simulink library "VCTlbx"  (R2018b)
settings: Solver=VariableStepAuto  StartTime=0.0  StopTime=10.0  RelTol=1e-3  EnableMultiTasking=on
undefined symbols (not defined in the file or in its folder): prefix, suffix
libraries: commrandsrc3 x3, powerlib_meascontrol x2, $bdroot x2, simulink x1
settings Model: Creator=Ulysses  LastModifiedBy=bernardu
settings DataIOCC: LimitDataPoints=on
settings OptimizationCC: LifeSpan=inf
settings DebuggingCC: AllowSymbolicDim=off  SFUnexpectedBacktrackingDiag=warning  SFNoUnconditionalDefaultTransitionDiag=warning
settings ModelReferenceCC: PropagateSignalLabelsOutOfModel=off
settings SFSimCC: SimUseLocalCustomCode=off
settings RTWCC: RTWUseLocalCustomCode=off
settings CodeAppCC: StateflowObjectComments=on
settings GRTTargetCC: TargetLangStandard=C89/C90 (ANSI)
settings ConfigComp: CovMetricSettings=dw  CovHtmlReporting=on  CovSaveCumulativeToWorkspaceVar=on  CovSaveSingleToWorkspaceVar=on  CovExternalEMLEnable=off

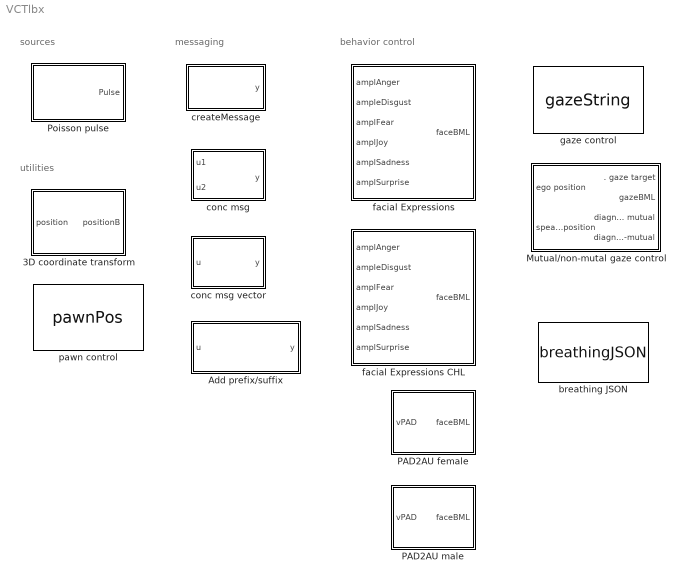
== system VCTlbx ==
  note: utilities
  note: sources
  note: behavior control
  note: messaging
  3D coordinate transform : Subsystem  mask(3D coordinate transform){zeroA=[], zeroB=[], minmaxXA=[], minmaxXB=[], minmaxYA=[], minmaxYB=[], minmaxZA=[], minmaxZB=[]}
      mask prompts: zeroA "center point input [3D]"; zeroB "center point output [3D]"; minmaxXA "min/max X input [2D]"; minmaxXB "min/max X output [2D]"; minmaxYA "min/max Y input [2D]"; minmaxYB "min/max Y output [2D]"; minmaxZA "min/max Z input [2D]"; minmaxZB "min/max Z output [2D]"
      mask help: Transform 3D coordinates from scale and center to another.
      mask TypeOptions zeroA: zeroA/zeroA
      mask TypeOptions zeroB: zeroB/zeroB
      mask TypeOptions minmaxXA: minmaxXA/minmaxXA
      mask TypeOptions minmaxXB: minmaxXB/minmaxXB
      mask TypeOptions minmaxYA: minmaxYA/minmaxYA
      mask TypeOptions minmaxYB: minmaxYB/minmaxYB
      mask TypeOptions minmaxZA: minmaxZA/minmaxZA
      mask TypeOptions minmaxZB: minmaxZB/minmaxZB
  Add prefix/suffix : MATLAB Function  TreatAsAtomicUnit=on  mask(Prefix/suffix message){paramPrefix=<?xml version="1.0" ?><act><bml>, paramSuffix=</bml></act>}
  Mutual/non-mutal gaze control : Subsystem  Description=|  mask(Mutual/non-mutal randomized gaze){PoissonParameterMutual=5, PoissonParameterNonMutual=5, paramVarianceVertical=pi/10, paramExtent=.3, paramVarianceHorizontal=pi/2}
      | this block implements an oscillation between two Poisson processes; one for mutual and 
      | one for non-mutual gaze
      mask prompts: PoissonParameterMutual "Poisson parameter (Lambda) for mutual gaze:"; PoissonParameterNonMutual "Poisson parameter (Lambda) for non-mutual gaze:"; paramVarianceVertical "Variance vertical"; paramExtent "Extent [0...1]"; paramVarianceHorizontal "Variance horizontal"
      mask help:
      | this block implements an oscillation between two Poisson processes; one for mutual and
      | one for non-mutual gaze
      mask TypeOptions PoissonParameterMutual: Poisson social Gaze/PoissonParameterMutual
      mask TypeOptions PoissonParameterNonMutual: Poisson social Gaze/PoissonParameterNonMutual
      mask TypeOptions paramVarianceVertical: randomGaze1/RN vert/Variance
      mask TypeOptions paramExtent: Extent/Value
      mask TypeOptions paramVarianceHorizontal: randomGaze1/RN horiz/Variance
  PAD2AU female : Subsystem  mask(PAD to face BML (female)){gainAU_1=[-0.086 -0.001 -0.062], gainAU_2=[0.015 +0.018 +0.104], gainAU_4=[-0.067 -0.017 +0.078], gainAU_5=[0.003 +0.120 -0.017], gainAU_6=[-0.009 -0.012 +0.036], gainAU_7=[0.004 -0.021 +0.040], gainAU_9=[-0.007 +0.001 +0.086], gainAU_10=[-0.089 -0.007 +0.028], gainAU_11=[0.000 -0.017 +0.028], gainAU_12=[0.114 -0.009 +0.013], gainAU_13=[0.063 -0.011 +0.033], gainAU_14=[0.049 -0.025 +0.054], gainAU_15=[-0.073 -0.008 +0.035], gainAU_16=[-0.048 +0.049 +0.006], gainAU_17=[-0.071 -0.005 +0.023], gainAU_18=[0.013 -0.033 +0.041], gainAU_20=[-0.009 -0.010 +0.029], gainAU_22=[0.057 +0.013 -0.002], gainAU_23=[0.009 -0.007 +0.050], gainAU_24=[-0.016 -0.042 +0.041], gainAU_25=[0.157 +0.100 +0.095], gainAU_26=[0.041 -0.022 +0.081], gainAU_27=[0.060 +0.079 +0.127], gainAD_28=[0.017 -0.031 +0.052], gainAD_29=[-0.001 -0.010 +0.051], gainAU_30=[-0.005 -0.003 -0.004], gainAU_31=[-0.016 +0.013 +0.052], gainAU_32=[-0.012 -0.044 +0.006], gainAU_33=[-0.017 -0.006 +0.032], gainAD_34=[0.009 -0.028 +0.035], gainAD_35=[0.000 -0.019 +0.044], gainAU_38=[-0.023 -0.018 +0.050], gainAU_39=[-0.004 -0.024 +0.034], gainAU_43=[-0.019 -0.131 +0.076]}
      mask prompts: gainAU_1 "gain for AU_1"; gainAU_2 "gain for AU_2"; gainAU_4 "gain for AU_4"; gainAU_5 "gain for AU_5"; gainAU_6 "gain for AU_6"; gainAU_7 "gain for AU_7"; gainAU_9 "gain for AU_9"; gainAU_10 "gain for AU_10"; gainAU_11 "gain for AU_11"; gainAU_12 "gain for AU_12"; gainAU_13 "gain for AU_13"; gainAU_14 "gain for AU_14"; gainAU_15 "gain for AU_15"; gainAU_16 "gain for AU_16"; gainAU_17 "gain for AU_17"; gainAU_18 "gain for AU_18"; gainAU_20 "gain for AU_20"; gainAU_22 "gain for AU_22"; gainAU_23 "gain for AU_23"; gainAU_24 "gain for AU_24"; gainAU_25 "gain for AU_25"; gainAU_26 "gain for AU_26"; gainAU_27 "gain for AU_27"; gainAD_28 "gain for AD_28"; gainAD_29 "gain for AD_29"; gainAU_30 "gain for AU_30"; gainAU_31 "gain for AU_31"; gainAU_32 "gain for AU_32"; gainAU_33 "gain for AU_33"; gainAD_34 "gain for AD_34"; gainAD_35 "gain for AD_35"; gainAU_38 "gain for AU_38"; gainAU_39 "gain for AU_39"; gainAU_43 "gain for AU_43"
      mask help:
      | Creates a BML message from Pleasure Arousal Dominance input. Mappings are based on:
      | Hana Boukricha, Ipke Wachsmuth, Andrea Hofstatter, and Karl Grammer. 2009. Pleasure-arousal-dominance driven facial expression simulation. 2009 3rd International Conference on Affective Computing and Intelligent Interaction and Workshops, IEEE, 1–7. http://doi.org/10.1109/ACII.2009.5349579
      mask TypeOptions gainAU_1: gainAU_1/Gain
      mask TypeOptions gainAU_2: gainAU_2/Gain
      mask TypeOptions gainAU_4: gainAU_4/Gain
      mask TypeOptions gainAU_5: gainAU_5/Gain
      mask TypeOptions gainAU_6: gainAU_6/Gain
      mask TypeOptions gainAU_7: gainAU_7/Gain
      mask TypeOptions gainAU_9: gainAU_9/Gain
      mask TypeOptions gainAU_10: gainAU_10/Gain
      mask TypeOptions gainAU_11: gainAU_11/Gain
      mask TypeOptions gainAU_12: gainAU_12/Gain
      mask TypeOptions gainAU_13: gainAU_13/Gain
      mask TypeOptions gainAU_14: gainAU_14/Gain
      mask TypeOptions gainAU_15: gainAU_15/Gain
      mask TypeOptions gainAU_16: gainAU_16/Gain
      mask TypeOptions gainAU_17: gainAU_17/Gain
      mask TypeOptions gainAU_18: gainAU_18/Gain
      mask TypeOptions gainAU_20: gainAU_20/Gain
      mask TypeOptions gainAU_22: gainAU_22/Gain
      mask TypeOptions gainAU_23: gainAU_23/Gain
      mask TypeOptions gainAU_24: gainAU_24/Gain
      mask TypeOptions gainAU_25: gainAU_25/Gain
      mask TypeOptions gainAU_26: gainAU_26/Gain
      mask TypeOptions gainAU_27: gainAU_27/Gain
      mask TypeOptions gainAD_28: gainAD_28/Gain
      mask TypeOptions gainAD_29: gainAD_29/Gain
      mask TypeOptions gainAU_30: gainAU_30/Gain
      mask TypeOptions gainAU_31: gainAU_31/Gain
      mask TypeOptions gainAU_32: gainAU_32/Gain
      mask TypeOptions gainAU_33: gainAU_33/Gain
      mask TypeOptions gainAD_34: gainAD_34/Gain
      mask TypeOptions gainAD_35: gainAD_35/Gain
      mask TypeOptions gainAU_38: gainAU_38/Gain
      mask TypeOptions gainAU_39: gainAU_39/Gain
      mask TypeOptions gainAU_43: gainAU_43/Gain
  PAD2AU male : Subsystem  mask(PAD to face BML (male)){gainAU_1=[0.003 -0.002 -0.016 ], gainAU_2=[-0.002 +0.010 -0.030], gainAU_27=[-0.016 +0.034 +0.019], gainAU_26=[-0.002 +0.049 -0.006], gainAU_6=[-0.008 +0.009 +0.004], gainAU_18=[0.002 +0.004 +0.014 ], gainAU_22=[0.007 +0.025 +0.006 ], gainAU_14=[0.003 +0.009 -0.002 ], gainAU_17=[-0.010 +0.017 +0.000], gainAU_10=[-0.053 +0.026 +0.014], gainAU_5=[-0.003 +0.032 -0.000], gainAU_43=[-0.021 -0.037 -0.011], gainAU_4=[-0.036 +0.022 +0.019], gainAU_9=[-0.008 +0.006 +0.005], gainAU_39=[-0.004 +0.004 -0.008], gainAU_38=[-0.010 +0.008 +0.005], gainAU_25=[-0.023 +0.058 +0.008], gainAU_24=[-0.004 -0.003 -0.007], gainAU_23=[-0.011 +0.009 -0.007], gainAU_19=[-0.004 +0.003 +0.001], gainAU_13=[0.039 +0.015 -0.004 ], gainAU_7=[-0.005 -0.001 +0.009], gainAU_12=[0.057 +0.009 -0.019 ], gainAU_11=[-0.008 +0.009 +0.001], gainAU_15=[-0.046 -0.002 -0.003], gainAU_16=[-0.014 +0.016 -0.002], gainAU_20=[-0.026 +0.010 -0.002]}
      mask prompts: gainAU_1 "gain for AU_1"; gainAU_2 "gain for AU_2"; gainAU_27 "gain for AU_27"; gainAU_26 "gain for AU_26"; gainAU_6 "gain for AU_6"; gainAU_18 "gain for AU_18"; gainAU_22 "gain for AU_22"; gainAU_14 "gain for AU_14"; gainAU_17 "gain for AU_17"; gainAU_10 "gain for AU_10"; gainAU_5 "gain for AU_5"; gainAU_43 "gain for AU_43"; gainAU_4 "gain for AU_4"; gainAU_9 "gain for AU_9"; gainAU_39 "gain for AU_39"; gainAU_38 "gain for AU_38"; gainAU_25 "gain for AU_25"; gainAU_24 "gain for AU_24"; gainAU_23 "gain for AU_23"; gainAU_19 "gain for AU_19"; gainAU_13 "gain for AU_13"; gainAU_7 "gain for AU_7"; gainAU_12 "gain for AU_12"; gainAU_11 "gain for AU_11"; gainAU_15 "gain for AU_15"; gainAU_16 "gain for AU_16"; gainAU_20 "gain for AU_20"
      mask help:
      | Creates a BML message from Pleasure Arousal Dominance input. Mappings are based on:
      | Hana Boukricha, Ipke Wachsmuth, Andrea Hofstatter, and Karl Grammer. 2009. Pleasure-arousal-dominance driven facial expression simulation. 2009 3rd International Conference on Affective Computing and Intelligent Interaction and Workshops, IEEE, 1–7. http://doi.org/10.1109/ACII.2009.5349579
      mask TypeOptions gainAU_1: gainAU_1/Gain
      mask TypeOptions gainAU_2: gainAU_2/Gain
      mask TypeOptions gainAU_27: gainAU_27/Gain
      mask TypeOptions gainAU_26: gainAU_26/Gain
      mask TypeOptions gainAU_6: gainAU_6/Gain
      mask TypeOptions gainAU_18: gainAU_18/Gain
      mask TypeOptions gainAU_22: gainAU_22/Gain
      mask TypeOptions gainAU_14: gainAU_14/Gain
      mask TypeOptions gainAU_17: gainAU_17/Gain
      mask TypeOptions gainAU_10: gainAU_10/Gain
      mask TypeOptions gainAU_5: gainAU_5/Gain
      mask TypeOptions gainAU_43: gainAU_43/Gain
      mask TypeOptions gainAU_4: gainAU_4/Gain
      mask TypeOptions gainAU_9: gainAU_9/Gain
      mask TypeOptions gainAU_39: gainAU_39/Gain
      mask TypeOptions gainAU_38: gainAU_38/Gain
      mask TypeOptions gainAU_25: gainAU_25/Gain
      mask TypeOptions gainAU_24: gainAU_24/Gain
      mask TypeOptions gainAU_23: gainAU_23/Gain
      mask TypeOptions gainAU_19: gainAU_19/Gain
      mask TypeOptions gainAU_13: gainAU_13/Gain
      mask TypeOptions gainAU_7: gainAU_7/Gain
      mask TypeOptions gainAU_12: gainAU_12/Gain
      mask TypeOptions gainAU_11: gainAU_11/Gain
      mask TypeOptions gainAU_15: gainAU_15/Gain
      mask TypeOptions gainAU_16: gainAU_16/Gain
      mask TypeOptions gainAU_20: gainAU_20/Gain
  Poisson pulse : Subsystem  mask(Poisson pulse){PoissonParameter=3}
      mask prompts: PoissonParameter "Poisson parameter (Lambda):"
      mask help: Generates a pulse train with Poisson distributed delays.
      mask TypeOptions PoissonParameter: triggered Poisson/Poisson numbers/PoissonParameter
  breathing JSON : S-Function  FunctionName=breathingJSON  Parameters=double(charname)  SFunctionDeploymentMode=off  EnableBusSupport=off  mask(Send JSON formatted breathing blendshape control){charname='FuseCharacter'}
      mask prompts: charname "Character Name"
      mask help:
      | Send JSON with the following format:
      | {
      |    "blendshape_ctrl":{
      |       "blendshapes_names":[
      |          "Tops_BreatheChest",
      |          "Tops_BreatheStomach"
      |       ],
      |       "blendshapes_weights":[
      |          <thx>,
      |          <abd>
      |       ],
      |       "mesh":"Tops"
      |    },
      |    "character":"FuseCharacter",
      |    "joint_rotation":{
      |       "name":"Hips/Spine/Spine1/Spine2/Neck/Head",
      |       "quaternion":[
      |          <x>,
      |          <y>,
      |          <z>,
      |          <w>
      |       ]
      |    }
      | }
      mask Display:
      | port_label('input', 1, 'thx')
      | port_label('input', 2, 'abd')
      | port_label('input', 3, 'neck')
      | port_label('output', 1, 'JSON')
      | disp('{}')
  conc msg : MATLAB Function  TreatAsAtomicUnit=on  mask(Concatenate messages){}
      mask help: Concatenates all messages (represented as double arrays) into a single one. Max length of concatenated message is 2048.
  conc msg vector : MATLAB Function  TreatAsAtomicUnit=on  mask(Concatenate messages){}
      mask help: Concatenates all messages (represented as double arrays) into a single one. Max length of concatenated message is 2048.
  createMessage : MATLAB Function  TreatAsAtomicUnit=on  mask(createMessage){paramMessage=message}
      mask prompts: paramMessage "Message"
      mask help: Create double array message from input string. Max length = 2048. DO NOT USE QUOTES
  facial Expressions : Subsystem  mask(Categorical facial experssions){}
      mask help: Block to generate categorical facial expressions. Input is amplitude [0...1].
      mask Display:
      | port_label('input', 1, 'ampl. Anger');
      | port_label('input', 2, 'ampl. Disgust');
      | port_label('input', 3, 'ampl. Fear');
      | port_label('input', 4, 'ampl. Joy');
      | port_label('input', 5, 'ampl. Sadness');
      | port_label('input', 6, 'ampl. Surprise');
      | port_label('output', 1, 'faceBML');
  facial Expressions CHL : Subsystem  AncestorBlock=VCTlbx/facial Expressions  mask(Categorical facial experssions){}
      mask help: Block to generate categorical facial expressions. Input is amplitude [0...1].
      mask Display:
      | port_label('input', 1, 'ampl. Anger');
      | port_label('input', 2, 'ampl. Disgust');
      | port_label('input', 3, 'ampl. Fear');
      | port_label('input', 4, 'ampl. Joy');
      | port_label('input', 5, 'ampl. Sadness');
      | port_label('input', 6, 'ampl. Surprise');
      | port_label('output', 1, 'faceBML');
  gaze control : S-Function  FunctionName=gazeString  SFunctionDeploymentMode=off  EnableBusSupport=off  mask(gaze BML){}
      mask Display:
      | port_label('input', 1, 'xpos')
      | port_label('input', 2, 'ypos')
      | port_label('input', 3, 'zpos')
      | port_label('input', 4, 'extent')
      | port_label('output', 1, 'gaze BML')
  pawn control : S-Function  FunctionName=pawnPos  SFunctionDeploymentMode=off  EnableBusSupport=off
      mask Display:
      | port_label('input', 1, 'xpos')
      | port_label('input', 2, 'ypos')
      | port_label('input', 3, 'zpos')
      | port_label('output', 1, 'pawn SBM')

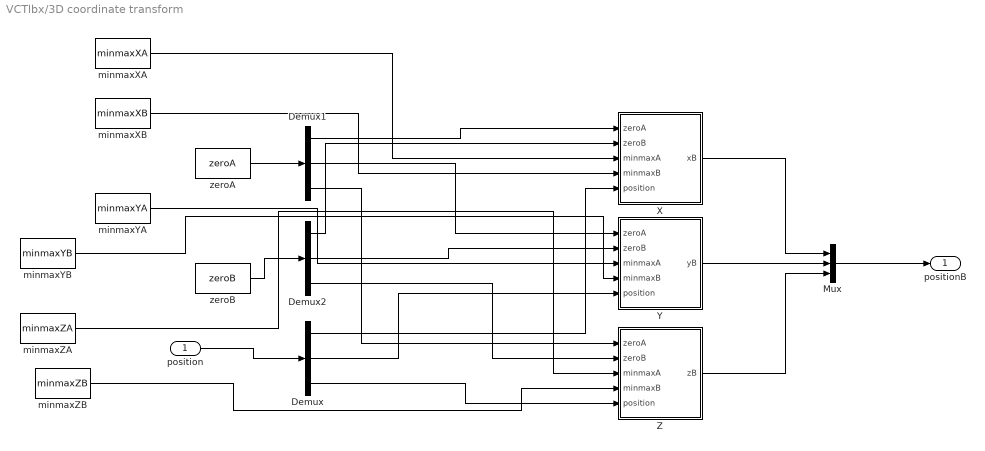
== system VCTlbx/3D coordinate transform ==
  position : Inport  PortDimensions=3
  Demux : Demux  Outputs=3
  Demux1 : Demux  Outputs=3
  Demux2 : Demux  Outputs=3
  Mux : Mux  Inputs=3
  X : Subsystem
  Y : Subsystem
  Z : Subsystem
  minmaxXA : Constant  Value=minmaxXA  VectorParams1D=off  mask{minmaxXA=minmaxXA}
      mask prompts: minmaxXA "min/max X input [2D]"
  minmaxXB : Constant  Value=minmaxXB  VectorParams1D=off  mask{minmaxXB=minmaxXB}
      mask prompts: minmaxXB "min/max X output [2D]"
  minmaxYA : Constant  Value=minmaxYA  VectorParams1D=off  mask{minmaxYA=minmaxYA}
      mask prompts: minmaxYA "min/max Y input [2D]"
  minmaxYB : Constant  Value=minmaxYB  VectorParams1D=off  mask{minmaxYB=minmaxYB}
      mask prompts: minmaxYB "min/max Y output [2D]"
  minmaxZA : Constant  Value=minmaxZA  VectorParams1D=off  mask{minmaxZA=minmaxZA}
      mask prompts: minmaxZA "min/max Z input [2D]"
  minmaxZB : Constant  Value=minmaxZB  VectorParams1D=off  mask{minmaxZB=minmaxZB}
      mask prompts: minmaxZB "min/max Z output [2D]"
  zeroA : Constant  Value=zeroA  VectorParams1D=off  mask{zeroA=zeroA}
      mask prompts: zeroA "center point input [3D]"
  zeroB : Constant  Value=zeroB  VectorParams1D=off  mask{zeroB=zeroB}
      mask prompts: zeroB "center point output [3D]"
  positionB : Outport
  wires:
  Demux/1 -> X/5(position)
  Demux1/3 -> Z/1(zeroA)
  Demux1/2 -> Y/1(zeroA)
  Demux2/1 -> X/2(zeroB)
  X/1(xB) -> Mux/1
  Demux/3 -> Z/5(position)
  Demux1/1 -> X/1(zeroA)
  position/1 -> Demux/1
  Demux/2 -> Y/5(position)
  Y/1(yB) -> Mux/2
  minmaxXA/1 -> X/3(minmaxA)
  Z/1(zB) -> Mux/3
  minmaxYB/1 -> Y/4(minmaxB)
  minmaxXB/1 -> X/4(minmaxB)
  Mux/1 -> positionB/1
  Demux2/3 -> Z/2(zeroB)
  zeroA/1 -> Demux1/1
  zeroB/1 -> Demux2/1
  minmaxZB/1 -> Z/4(minmaxB)
  Demux2/2 -> Y/2(zeroB)
  minmaxYA/1 -> Y/3(minmaxA)
  minmaxZA/1 -> Z/3(minmaxA)

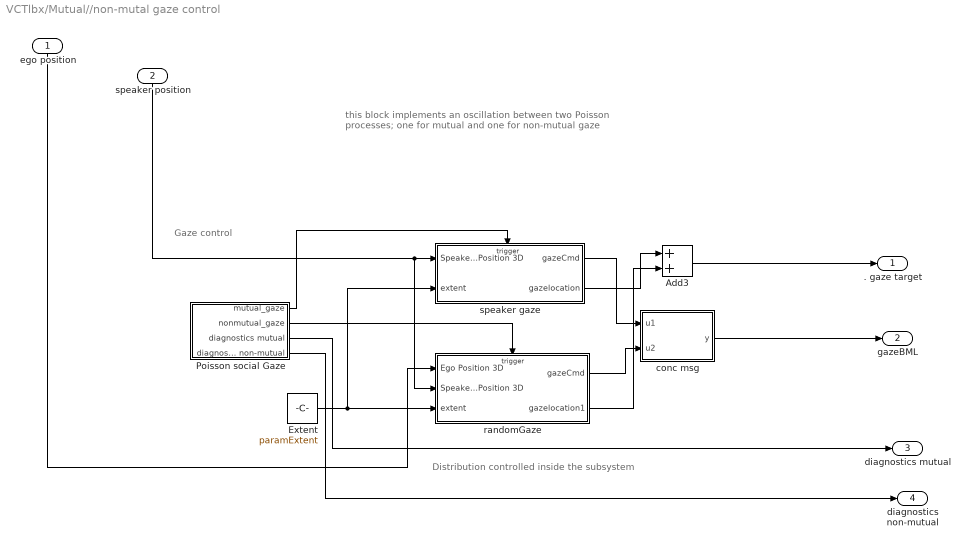
== system VCTlbx/Mutual//non-mutal gaze control ==
  note: Gaze control
  note: Distribution controlled inside the subsystem
  note: this block implements an oscillation
      | between two Poisson processes; one for mutual and
      | one for non-mutual gaze
  ego position : Inport
  speaker position : Inport  Port=2
  Add3 : Sum
  Extent : Constant  Value=paramExtent
  Poisson social Gaze : Subsystem  mask(Poisson pulse){PoissonParameterMutual=PoissonParameterMutual, PoissonParameterNonMutual=PoissonParameterNonMutual}
      mask prompts: PoissonParameterMutual "Poisson parameter (Lambda) for mutual gaze:"; PoissonParameterNonMutual "Poisson parameter (Lambda) for non-mutual gaze:"
      mask help: Generates a pulse train with Poisson distributed delays.
      mask TypeOptions PoissonParameterMutual: p mutual/Poisson numbers mutual/PoissonParameter
      mask TypeOptions PoissonParameterNonMutual: p nonmutual/Poisson numbers nonmutual/PoissonParameter
  conc msg : MATLAB Function  TreatAsAtomicUnit=on  mask(Concatenate messages){}
      mask help: Concatenates all messages (represented as double arrays) into a single one. Max length of concatenated message is 2048.
  randomGaze : Subsystem  TreatAsAtomicUnit=on
  speaker gaze : Subsystem  TreatAsAtomicUnit=on
  . gaze target : Outport
  gazeBML : Outport  Port=2
  diagnostics mutual : Outport  Port=3
  diagnostics non-mutual : Outport  Port=4
  wires:
  Poisson social Gaze/4(diagnostics non-mutual) -> diagnostics non-mutual/1
  Poisson social Gaze/3(diagnostics mutual) -> diagnostics mutual/1
  Add3/1 -> . gaze target/1
  Extent/1 -> randomGaze/3(extent), speaker gaze/2(extent)
  speaker gaze/2(gazelocation) -> Add3/1
  Poisson social Gaze/2(nonmutual_gaze) -> randomGaze/Trigger
  ego position/1 -> randomGaze/1(Ego Position 3D)
  randomGaze/1(gazeCmd) -> conc msg/2(u2)
  randomGaze/2(gazelocation1) -> Add3/2
  speaker position/1 -> speaker gaze/1("Speaker Position 3D "), randomGaze/2("Speaker Position 3D ")
  speaker gaze/1(gazeCmd) -> conc msg/1(u1)
  Poisson social Gaze/1(mutual_gaze) -> speaker gaze/Trigger
  conc msg/1(y) -> gazeBML/1

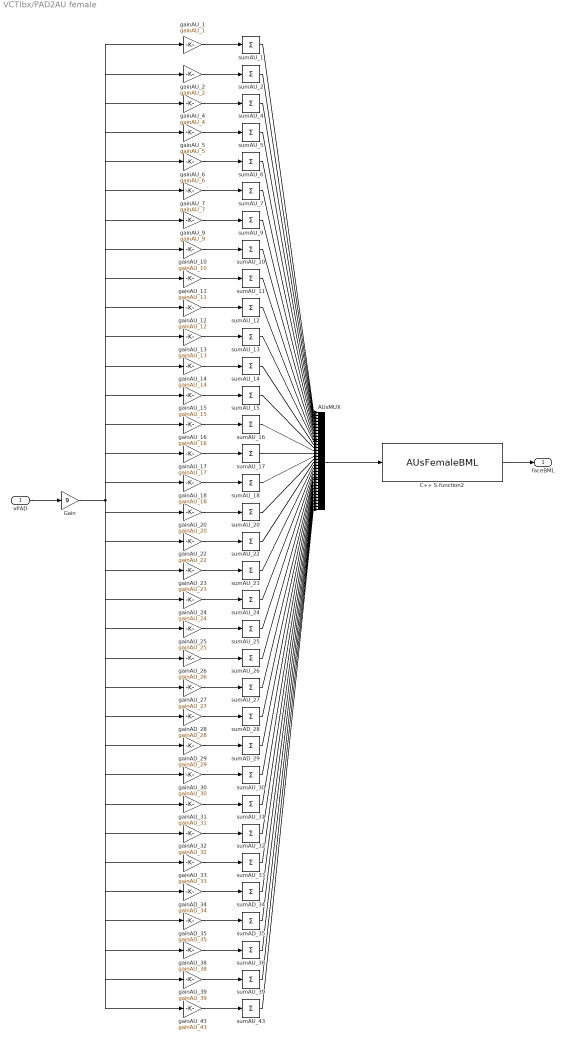
== system VCTlbx/PAD2AU female ==
  vPAD : Inport
  AUsMUX : Mux  Inputs=34
  C++ S-function2 : S-Function  FunctionName=AUsFemaleBML  SFunctionDeploymentMode=off  EnableBusSupport=off
  Gain : Gain  Gain=9
  gainAD_28 : Gain  Gain=gainAD_28
  gainAD_29 : Gain  Gain=gainAD_29
  gainAD_34 : Gain  Gain=gainAD_34
  gainAD_35 : Gain  Gain=gainAD_35
  gainAU_1 : Gain  Gain=gainAU_1
  gainAU_10 : Gain  Gain=gainAU_10
  gainAU_11 : Gain  Gain=gainAU_11
  gainAU_12 : Gain  Gain=gainAU_12
  gainAU_13 : Gain  Gain=gainAU_13
  gainAU_14 : Gain  Gain=gainAU_14
  gainAU_15 : Gain  Gain=gainAU_15
  gainAU_16 : Gain  Gain=gainAU_16
  gainAU_17 : Gain  Gain=gainAU_17
  gainAU_18 : Gain  Gain=gainAU_18
  gainAU_2 : Gain  Gain=gainAU_2
  gainAU_20 : Gain  Gain=gainAU_20
  gainAU_22 : Gain  Gain=gainAU_22
  gainAU_23 : Gain  Gain=gainAU_23
  gainAU_24 : Gain  Gain=gainAU_24
  gainAU_25 : Gain  Gain=gainAU_25
  gainAU_26 : Gain  Gain=gainAU_26
  gainAU_27 : Gain  Gain=gainAU_27
  gainAU_30 : Gain  Gain=gainAU_30
  gainAU_31 : Gain  Gain=gainAU_31
  gainAU_32 : Gain  Gain=gainAU_32
  gainAU_33 : Gain  Gain=gainAU_33
  gainAU_38 : Gain  Gain=gainAU_38
  gainAU_39 : Gain  Gain=gainAU_39
  gainAU_4 : Gain  Gain=gainAU_4
  gainAU_43 : Gain  Gain=gainAU_43
  gainAU_5 : Gain  Gain=gainAU_5
  gainAU_6 : Gain  Gain=gainAU_6
  gainAU_7 : Gain  Gain=gainAU_7
  gainAU_9 : Gain  Gain=gainAU_9
  sumAD_{28..29,34..35} (4 alike) : Sum  Inputs=+
  sumAU_{1..2,4..7,9..18,20,22..27,30..33,38..39,43} (30 alike) : Sum  Inputs=+
  faceBML : Outport
  wires:
  AUsMUX/1 -> C++ S-function2/1
  sumAU_6/1 -> AUsMUX/5
  gainAU_6/1 -> sumAU_6/1
  gainAU_7/1 -> sumAU_7/1
  sumAU_9/1 -> AUsMUX/7
  gainAU_9/1 -> sumAU_9/1
  sumAU_7/1 -> AUsMUX/6
  gainAU_10/1 -> sumAU_10/1
  sumAU_10/1 -> AUsMUX/8
  sumAU_14/1 -> AUsMUX/12
  gainAU_15/1 -> sumAU_15/1
  sumAU_15/1 -> AUsMUX/13
  gainAU_14/1 -> sumAU_14/1
  sumAU_16/1 -> AUsMUX/14
  gainAU_17/1 -> sumAU_17/1
  gainAU_16/1 -> sumAU_16/1
  sumAU_4/1 -> AUsMUX/3
  sumAU_2/1 -> AUsMUX/2
  gainAU_2/1 -> sumAU_2/1
  gainAU_4/1 -> sumAU_4/1
  sumAU_5/1 -> AUsMUX/4
  gainAU_5/1 -> sumAU_5/1
  gainAU_11/1 -> sumAU_11/1
  sumAU_11/1 -> AUsMUX/9
  gainAU_13/1 -> sumAU_13/1
  gainAU_12/1 -> sumAU_12/1
  sumAU_12/1 -> AUsMUX/10
  sumAU_13/1 -> AUsMUX/11
  sumAU_18/1 -> AUsMUX/16
  sumAU_17/1 -> AUsMUX/15
  gainAU_18/1 -> sumAU_18/1
  gainAU_20/1 -> sumAU_20/1
  sumAU_22/1 -> AUsMUX/18
  sumAU_20/1 -> AUsMUX/17
  gainAU_22/1 -> sumAU_22/1
  gainAU_23/1 -> sumAU_23/1
  sumAU_23/1 -> AUsMUX/19
  gainAU_24/1 -> sumAU_24/1
  sumAU_25/1 -> AUsMUX/21
  gainAU_26/1 -> sumAU_26/1
  gainAU_25/1 -> sumAU_25/1
  sumAU_24/1 -> AUsMUX/20
  gainAD_28/1 -> sumAD_28/1
  sumAU_26/1 -> AUsMUX/22
  gainAU_27/1 -> sumAU_27/1
  sumAU_27/1 -> AUsMUX/23
  sumAD_29/1 -> AUsMUX/25
  sumAD_28/1 -> AUsMUX/24
  gainAD_29/1 -> sumAD_29/1
  sumAU_31/1 -> AUsMUX/27
  sumAU_30/1 -> AUsMUX/26
  gainAU_31/1 -> sumAU_31/1
  gainAU_30/1 -> sumAU_30/1
  sumAU_32/1 -> AUsMUX/28
  gainAU_32/1 -> sumAU_32/1
  gainAU_33/1 -> sumAU_33/1
  sumAU_33/1 -> AUsMUX/29
  gainAD_34/1 -> sumAD_34/1
  sumAD_35/1 -> AUsMUX/31
  gainAU_38/1 -> sumAU_38/1
  gainAD_35/1 -> sumAD_35/1
  sumAU_38/1 -> AUsMUX/32
  sumAD_34/1 -> AUsMUX/30
  gainAU_39/1 -> sumAU_39/1
  sumAU_39/1 -> AUsMUX/33
  gainAU_43/1 -> sumAU_43/1
  sumAU_43/1 -> AUsMUX/34
  sumAU_1/1 -> AUsMUX/1
  Gain/1 -> gainAU_1/1, gainAU_2/1, gainAU_4/1, gainAU_5/1, gainAU_6/1, gainAU_7/1, gainAU_9/1, gainAU_10/1, gainAU_11/1, gainAU_12/1, gainAU_13/1, gainAU_14/1, gainAU_15/1, gainAU_16/1, gainAU_17/1, gainAU_18/1, gainAU_20/1, gainAU_22/1, gainAU_23/1, gainAU_24/1, gainAU_25/1, gainAU_26/1, gainAU_27/1, gainAD_28/1, gainAD_29/1, gainAU_30/1, gainAU_31/1, gainAU_32/1, gainAU_33/1, gainAD_34/1, gainAD_35/1, gainAU_38/1, gainAU_39/1, gainAU_43/1
  gainAU_1/1 -> sumAU_1/1
  vPAD/1 -> Gain/1
  C++ S-function2/1 -> faceBML/1

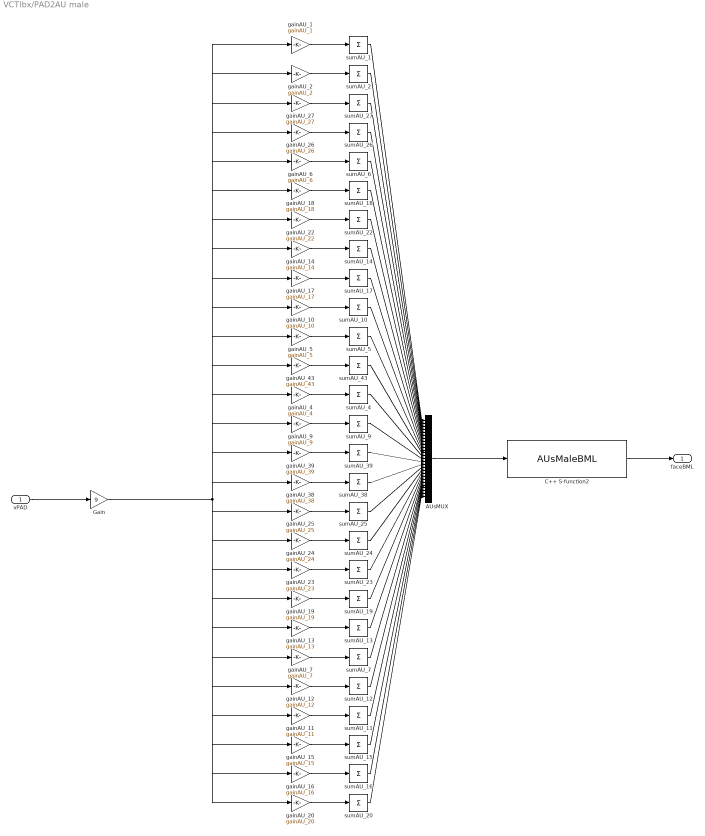
== system VCTlbx/PAD2AU male ==
  vPAD : Inport
  AUsMUX : Mux  Inputs=27
  C++ S-function2 : S-Function  FunctionName=AUsMaleBML  SFunctionDeploymentMode=off  EnableBusSupport=off
  Gain : Gain  Gain=9
  gainAU_1 : Gain  Gain=gainAU_1
  gainAU_10 : Gain  Gain=gainAU_10
  gainAU_11 : Gain  Gain=gainAU_11
  gainAU_12 : Gain  Gain=gainAU_12
  gainAU_13 : Gain  Gain=gainAU_13
  gainAU_14 : Gain  Gain=gainAU_14
  gainAU_15 : Gain  Gain=gainAU_15
  gainAU_16 : Gain  Gain=gainAU_16
  gainAU_17 : Gain  Gain=gainAU_17
  gainAU_18 : Gain  Gain=gainAU_18
  gainAU_19 : Gain  Gain=gainAU_19
  gainAU_2 : Gain  Gain=gainAU_2
  gainAU_20 : Gain  Gain=gainAU_20
  gainAU_22 : Gain  Gain=gainAU_22
  gainAU_23 : Gain  Gain=gainAU_23
  gainAU_24 : Gain  Gain=gainAU_24
  gainAU_25 : Gain  Gain=gainAU_25
  gainAU_26 : Gain  Gain=gainAU_26
  gainAU_27 : Gain  Gain=gainAU_27
  gainAU_38 : Gain  Gain=gainAU_38
  gainAU_39 : Gain  Gain=gainAU_39
  gainAU_4 : Gain  Gain=gainAU_4
  gainAU_43 : Gain  Gain=gainAU_43
  gainAU_5 : Gain  Gain=gainAU_5
  gainAU_6 : Gain  Gain=gainAU_6
  gainAU_7 : Gain  Gain=gainAU_7
  gainAU_9 : Gain  Gain=gainAU_9
  sumAU_{1..2,4..7,9..20,22..27,38..39,43} (27 alike) : Sum  Inputs=+
  faceBML : Outport
  wires:
  gainAU_17/1 -> sumAU_17/1
  gainAU_14/1 -> sumAU_14/1
  sumAU_14/1 -> AUsMUX/8
  sumAU_22/1 -> AUsMUX/7
  sumAU_26/1 -> AUsMUX/4
  gainAU_26/1 -> sumAU_26/1
  gainAU_6/1 -> sumAU_6/1
  sumAU_6/1 -> AUsMUX/5
  gainAU_18/1 -> sumAU_18/1
  sumAU_18/1 -> AUsMUX/6
  gainAU_22/1 -> sumAU_22/1
  Gain/1 -> gainAU_1/1, gainAU_2/1, gainAU_27/1, gainAU_26/1, gainAU_6/1, gainAU_18/1, gainAU_22/1, gainAU_14/1, gainAU_17/1, gainAU_10/1, gainAU_5/1, gainAU_43/1, gainAU_4/1, gainAU_9/1, gainAU_39/1, gainAU_38/1, gainAU_25/1, gainAU_24/1, gainAU_23/1, gainAU_19/1, gainAU_13/1, gainAU_7/1, gainAU_12/1, gainAU_11/1, gainAU_15/1, gainAU_16/1, gainAU_20/1
  gainAU_15/1 -> sumAU_15/1
  gainAU_11/1 -> sumAU_11/1
  sumAU_11/1 -> AUsMUX/24
  AUsMUX/1 -> C++ S-function2/1
  sumAU_24/1 -> AUsMUX/18
  gainAU_24/1 -> sumAU_24/1
  gainAU_7/1 -> sumAU_7/1
  sumAU_7/1 -> AUsMUX/22
  gainAU_12/1 -> sumAU_12/1
  sumAU_12/1 -> AUsMUX/23
  sumAU_19/1 -> AUsMUX/20
  gainAU_13/1 -> sumAU_13/1
  sumAU_13/1 -> AUsMUX/21
  gainAU_19/1 -> sumAU_19/1
  gainAU_43/1 -> sumAU_43/1
  sumAU_43/1 -> AUsMUX/12
  gainAU_10/1 -> sumAU_10/1
  sumAU_10/1 -> AUsMUX/10
  sumAU_17/1 -> AUsMUX/9
  gainAU_5/1 -> sumAU_5/1
  sumAU_5/1 -> AUsMUX/11
  gainAU_16/1 -> sumAU_16/1
  sumAU_16/1 -> AUsMUX/26
  sumAU_15/1 -> AUsMUX/25
  sumAU_23/1 -> AUsMUX/19
  gainAU_23/1 -> sumAU_23/1
  gainAU_20/1 -> sumAU_20/1
  sumAU_20/1 -> AUsMUX/27
  sumAU_1/1 -> AUsMUX/1
  gainAU_1/1 -> sumAU_1/1
  sumAU_2/1 -> AUsMUX/2
  sumAU_27/1 -> AUsMUX/3
  gainAU_2/1 -> sumAU_2/1
  gainAU_27/1 -> sumAU_27/1
  sumAU_25/1 -> AUsMUX/17
  sumAU_38/1 -> AUsMUX/16
  gainAU_38/1 -> sumAU_38/1
  gainAU_25/1 -> sumAU_25/1
  sumAU_4/1 -> AUsMUX/13
  gainAU_4/1 -> sumAU_4/1
  gainAU_9/1 -> sumAU_9/1
  sumAU_9/1 -> AUsMUX/14
  sumAU_39/1 -> AUsMUX/15
  gainAU_39/1 -> sumAU_39/1
  C++ S-function2/1 -> faceBML/1
  vPAD/1 -> Gain/1

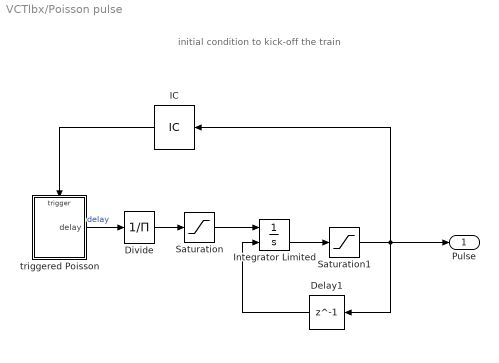
== system VCTlbx/Poisson pulse ==
  note: initial condition to kick-off the train
  Delay1 : Delay  DelayLength=1
  Divide : Product  Inputs=/
  IC : InitialCondition
  Integrator Limited : Integrator  ExternalReset=rising  LimitOutput=on  UpperSaturationLimit=1  LowerSaturationLimit=0  ShowSaturationPort=on
  Saturation : Saturate  UpperLimit=100  LowerLimit=0
  Saturation1 : Saturate  UpperLimit=1  LowerLimit=0
  triggered Poisson : Subsystem
  Pulse : Outport
  wires:
  triggered Poisson/1(delay) -> Divide/1  "delay"
  Delay1/1 -> Integrator Limited/2
  Divide/1 -> Saturation/1
  Saturation/1 -> Integrator Limited/1
  Integrator Limited/2 -> Saturation1/1
  IC/1 -> triggered Poisson/Trigger
  Saturation1/1 -> IC/1, Delay1/1, Pulse/1

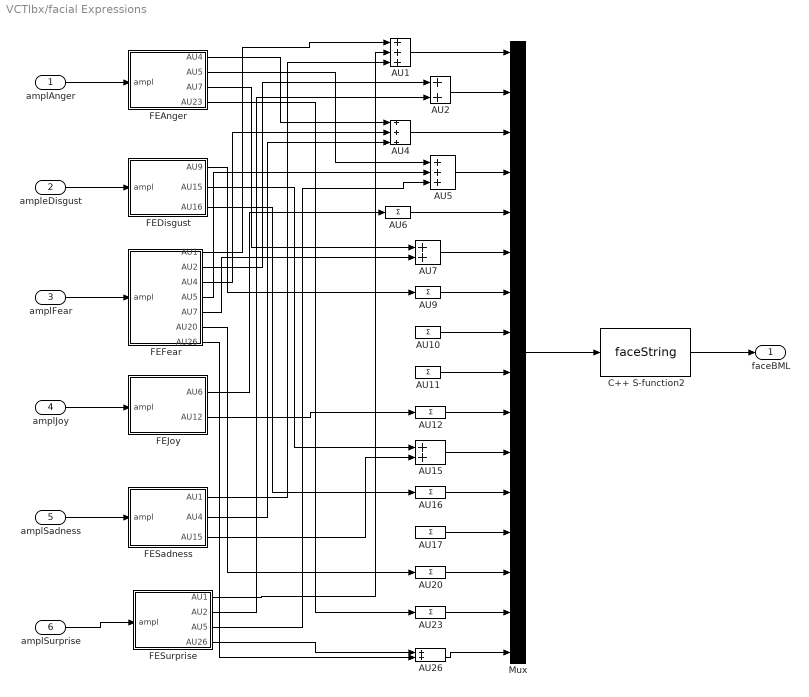
== system VCTlbx/facial Expressions ==
  amplAnger : Inport
  ampleDisgust : Inport  Port=2
  amplFear : Inport  Port=3
  amplJoy : Inport  Port=4
  amplSadness : Inport  Port=5
  amplSurprise : Inport  Port=6
  AU1 : Sum  Inputs=+++
  AU{6,9..12,16..17,20,23} (9 alike) : Sum  Inputs=+
  AU{2,7,15,26} (4 alike) : Sum
  AU4 : Sum  Inputs=+++
  AU5 : Sum  Inputs=+++
  C++ S-function2 : S-Function  FunctionName=faceString  SFunctionDeploymentMode=off  EnableBusSupport=off
  FEAnger : MATLAB Function  TreatAsAtomicUnit=on
  FEDisgust : MATLAB Function  TreatAsAtomicUnit=on
  FEFear : MATLAB Function  TreatAsAtomicUnit=on
  FEJoy : MATLAB Function  TreatAsAtomicUnit=on
  FESadness : MATLAB Function  TreatAsAtomicUnit=on
  FESurprise : MATLAB Function  TreatAsAtomicUnit=on
  Mux : Mux  Inputs=16
  faceBML : Outport
  wires:
  amplSurprise/1 -> FESurprise/1(ampl)
  C++ S-function2/1 -> faceBML/1
  amplFear/1 -> FEFear/1(ampl)
  amplAnger/1 -> FEAnger/1(ampl)
  ampleDisgust/1 -> FEDisgust/1(ampl)
  amplJoy/1 -> FEJoy/1(ampl)
  amplSadness/1 -> FESadness/1(ampl)
  FEFear/1(AU1) -> AU1/1
  FESurprise/1(AU1) -> AU1/2
  FESurprise/2(AU2) -> AU2/2
  FEJoy/1(AU6) -> AU6/1
  FESurprise/3(AU5) -> AU5/3
  FEAnger/3(AU7) -> AU7/1
  FEDisgust/2(AU15) -> AU15/1
  FESurprise/4(AU26) -> AU26/1
  FEJoy/2(AU12) -> AU12/1
  FEDisgust/3(AU16) -> AU16/1
  AU1/1 -> Mux/1
  AU2/1 -> Mux/2
  AU4/1 -> Mux/3
  AU5/1 -> Mux/4
  AU6/1 -> Mux/5
  AU7/1 -> Mux/6
  AU9/1 -> Mux/7
  AU10/1 -> Mux/8
  AU11/1 -> Mux/9
  AU12/1 -> Mux/10
  AU17/1 -> Mux/13
  AU20/1 -> Mux/14
  AU26/1 -> Mux/16
  Mux/1 -> C++ S-function2/1
  AU23/1 -> Mux/15
  FEAnger/1(AU4) -> AU4/1
  FEAnger/2(AU5) -> AU5/1
  FEAnger/4(AU23) -> AU23/1
  AU15/1 -> Mux/11
  AU16/1 -> Mux/12
  FESadness/3(AU15) -> AU15/2
  FESadness/2(AU4) -> AU4/3
  FESadness/1(AU1) -> AU1/3
  FEFear/6(AU20) -> AU20/1
  FEFear/7(AU26) -> AU26/2
  FEFear/5(AU7) -> AU7/2
  FEFear/4(AU5) -> AU5/2
  FEFear/3(AU4) -> AU4/2
  FEFear/2(AU2) -> AU2/1
  FEDisgust/1(AU9) -> AU9/1

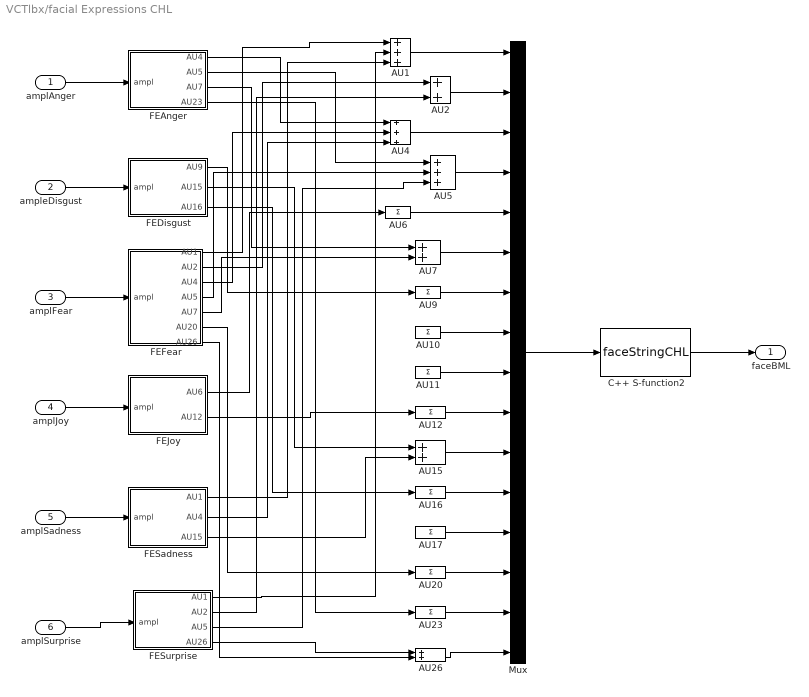
== system VCTlbx/facial Expressions CHL ==
  amplAnger : Inport
  ampleDisgust : Inport  Port=2
  amplFear : Inport  Port=3
  amplJoy : Inport  Port=4
  amplSadness : Inport  Port=5
  amplSurprise : Inport  Port=6
  AU1 : Sum  Inputs=+++
  AU{6,9..12,16..17,20,23} (9 alike) : Sum  Inputs=+
  AU{2,7,15,26} (4 alike) : Sum
  AU4 : Sum  Inputs=+++
  AU5 : Sum  Inputs=+++
  C++ S-function2 : S-Function  FunctionName=faceStringCHL  SFunctionDeploymentMode=off  EnableBusSupport=off
  FEAnger : MATLAB Function  TreatAsAtomicUnit=on
  FEDisgust : MATLAB Function  TreatAsAtomicUnit=on
  FEFear : MATLAB Function  TreatAsAtomicUnit=on
  FEJoy : MATLAB Function  TreatAsAtomicUnit=on
  FESadness : MATLAB Function  TreatAsAtomicUnit=on
  FESurprise : MATLAB Function  TreatAsAtomicUnit=on
  Mux : Mux  Inputs=16
  faceBML : Outport
  wires:
  amplSurprise/1 -> FESurprise/1(ampl)
  C++ S-function2/1 -> faceBML/1
  amplFear/1 -> FEFear/1(ampl)
  amplAnger/1 -> FEAnger/1(ampl)
  ampleDisgust/1 -> FEDisgust/1(ampl)
  amplJoy/1 -> FEJoy/1(ampl)
  amplSadness/1 -> FESadness/1(ampl)
  FEFear/1(AU1) -> AU1/1
  FESurprise/1(AU1) -> AU1/2
  FESurprise/2(AU2) -> AU2/2
  FEJoy/1(AU6) -> AU6/1
  FESurprise/3(AU5) -> AU5/3
  FEAnger/3(AU7) -> AU7/1
  FEDisgust/2(AU15) -> AU15/1
  FESurprise/4(AU26) -> AU26/1
  FEJoy/2(AU12) -> AU12/1
  FEDisgust/3(AU16) -> AU16/1
  AU1/1 -> Mux/1
  AU2/1 -> Mux/2
  AU4/1 -> Mux/3
  AU5/1 -> Mux/4
  AU6/1 -> Mux/5
  AU7/1 -> Mux/6
  AU9/1 -> Mux/7
  AU10/1 -> Mux/8
  AU11/1 -> Mux/9
  AU12/1 -> Mux/10
  AU17/1 -> Mux/13
  AU20/1 -> Mux/14
  AU26/1 -> Mux/16
  Mux/1 -> C++ S-function2/1
  AU23/1 -> Mux/15
  FEAnger/1(AU4) -> AU4/1
  FEAnger/2(AU5) -> AU5/1
  FEAnger/4(AU23) -> AU23/1
  AU15/1 -> Mux/11
  AU16/1 -> Mux/12
  FESadness/3(AU15) -> AU15/2
  FESadness/2(AU4) -> AU4/3
  FESadness/1(AU1) -> AU1/3
  FEFear/6(AU20) -> AU20/1
  FEFear/7(AU26) -> AU26/2
  FEFear/5(AU7) -> AU7/2
  FEFear/4(AU5) -> AU5/2
  FEFear/3(AU4) -> AU4/2
  FEFear/2(AU2) -> AU2/1
  FEDisgust/1(AU9) -> AU9/1

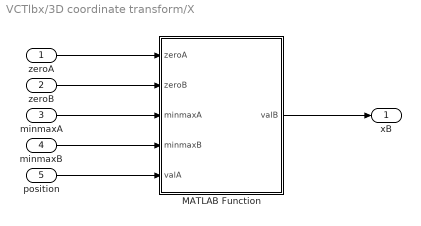
== system VCTlbx/3D coordinate transform/X ==
  zeroA : Inport
  zeroB : Inport  Port=2
  minmaxA : Inport  Port=3  PortDimensions=2
  minmaxB : Inport  Port=4  PortDimensions=2
  position : Inport  Port=5
  MATLAB Function : MATLAB Function  TreatAsAtomicUnit=on
  xB : Outport
  wires:
  MATLAB Function/1(valB) -> xB/1
  zeroA/1 -> MATLAB Function/1(zeroA)
  position/1 -> MATLAB Function/5(valA)
  zeroB/1 -> MATLAB Function/2(zeroB)
  minmaxA/1 -> MATLAB Function/3(minmaxA)
  minmaxB/1 -> MATLAB Function/4(minmaxB)

== system VCTlbx/3D coordinate transform/Y ==
  zeroA : Inport
  zeroB : Inport  Port=2
  minmaxA : Inport  Port=3  PortDimensions=2
  minmaxB : Inport  Port=4  PortDimensions=2
  position : Inport  Port=5
  MATLAB Function : MATLAB Function  TreatAsAtomicUnit=on
  yB : Outport
  wires:
  MATLAB Function/1(valB) -> yB/1
  zeroA/1 -> MATLAB Function/1(zeroA)
  position/1 -> MATLAB Function/5(valA)
  zeroB/1 -> MATLAB Function/2(zeroB)
  minmaxA/1 -> MATLAB Function/3(minmaxA)
  minmaxB/1 -> MATLAB Function/4(minmaxB)

== system VCTlbx/3D coordinate transform/Z ==
  zeroA : Inport
  zeroB : Inport  Port=2
  minmaxA : Inport  Port=3  PortDimensions=2
  minmaxB : Inport  Port=4  PortDimensions=2
  position : Inport  Port=5
  MATLAB Function : MATLAB Function  TreatAsAtomicUnit=on
  zB : Outport
  wires:
  MATLAB Function/1(valB) -> zB/1
  zeroA/1 -> MATLAB Function/1(zeroA)
  position/1 -> MATLAB Function/5(valA)
  zeroB/1 -> MATLAB Function/2(zeroB)
  minmaxA/1 -> MATLAB Function/3(minmaxA)
  minmaxB/1 -> MATLAB Function/4(minmaxB)

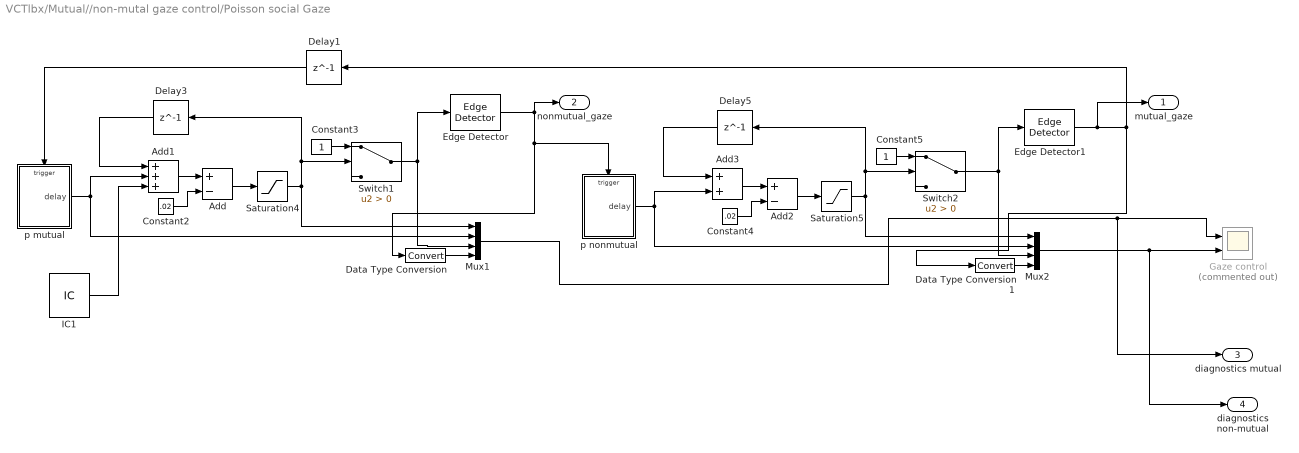
== system VCTlbx/Mutual//non-mutal gaze control/Poisson social Gaze ==
  Add : Sum  Inputs=+-
  Add1 : Sum  Inputs=+++
  Add2 : Sum  Inputs=+-
  Add3 : Sum
  Constant2 : Constant  Value=.02
  Constant3 : Constant
  Constant4 : Constant  Value=.02
  Constant5 : Constant
  Data Type Conversion : DataTypeConversion
  Data Type Conversion1 : DataTypeConversion
  Delay1 : Delay  DelayLength=1
  Delay3 : Delay  DelayLength=1
  Delay5 : Delay  DelayLength=1
  Edge Detector : powerlib_meascontrol/Logic/Edge Detector  model=Falling  ic=0  Ts=0
      settings: SourceProductName=Simscape Electrical  SourceProductBaseCode=PS
  Edge Detector1 : powerlib_meascontrol/Logic/Edge Detector  model=Falling  ic=0  Ts=0
      settings: SourceProductName=Simscape Electrical  SourceProductBaseCode=PS
  Gaze control : Scope  Commented=on  NumInputPorts=2
  IC1 : InitialCondition
  Mux1 : Mux
  Mux2 : Mux
  Saturation4 : Saturate  UpperLimit=inf  LowerLimit=0
  Saturation5 : Saturate  UpperLimit=inf  LowerLimit=0
  Switch1 : Switch  Criteria=u2 > Threshold
  Switch2 : Switch  Criteria=u2 > Threshold
  p mutual : Subsystem
  p nonmutual : Subsystem
  mutual_gaze : Outport
  nonmutual_gaze : Outport  Port=2
  diagnostics mutual : Outport  Port=3
  diagnostics non-mutual : Outport  Port=4
  wires:
  Delay1/1 -> p mutual/Trigger
  Edge Detector1/1 -> Data Type Conversion1/1, Delay1/1, mutual_gaze/1
  Data Type Conversion1/1 -> Mux2/4
  Data Type Conversion/1 -> Mux1/4
  Mux2/1 -> Gaze control/2, diagnostics non-mutual/1
  Mux1/1 -> Gaze control/1, diagnostics mutual/1
  Constant5/1 -> Switch2/1
  Switch2/1 -> Mux2/3, Edge Detector1/1
  p nonmutual/1(delay) -> Add3/2, Mux2/2
  Add2/1 -> Saturation5/1
  Add3/1 -> Add2/1
  Delay5/1 -> Add3/1
  Saturation5/1 -> Switch2/2, Delay5/1, Mux2/1
  Constant4/1 -> Add2/2
  Edge Detector/1 -> nonmutual_gaze/1, Data Type Conversion/1, p nonmutual/Trigger
  Constant3/1 -> Switch1/1
  Switch1/1 -> Edge Detector/1, Mux1/3
  p mutual/1(delay) -> Add1/2, Mux1/2
  IC1/1 -> Add1/3
  Add/1 -> Saturation4/1
  Add1/1 -> Add/1
  Delay3/1 -> Add1/1
  Saturation4/1 -> Switch1/2, Delay3/1, Mux1/1
  Constant2/1 -> Add/2

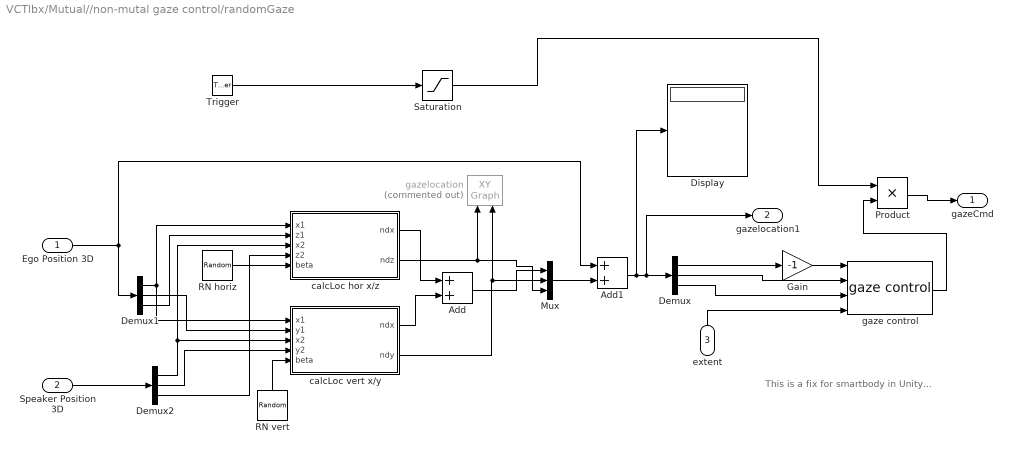
== system VCTlbx/Mutual//non-mutal gaze control/randomGaze ==
  note: This is a fix for smartbody in Unity...
  Ego Position 3D : Inport
  "Speaker Position 3D " : Inport  Port=2
  extent : Inport  Port=3
  Trigger : TriggerPort  TriggerType=either  VariantControl=Variant  ShowOutputPort=on
  Add : Sum
  Add1 : Sum
  Demux : Demux  Outputs=3
  Demux1 : Demux  Outputs=3
  Demux2 : Demux  Outputs=3
  Display : Display
  Gain : Gain  Gain=-1
  Mux : Mux  Inputs=3
  Product : Product
  RN horiz : RandomNumber  Variance=paramVarianceHorizontal
  RN vert : RandomNumber  Variance=paramVarianceVertical  Seed=1000
  Saturation : Saturate  UpperLimit=1  LowerLimit=0
  "calcLoc hor x/z " : MATLAB Function  TreatAsAtomicUnit=on
  calcLoc vert x/y : MATLAB Function  TreatAsAtomicUnit=on
  gaze control : $bdroot/gaze control  SFunctionModules=''
  gazelocation : simulink/Sinks/XY Graph  Commented=on  xmin=-10  xmax=10  ymin=-10  ymax=10  st=-1
  gazeCmd : Outport
  gazelocation1 : Outport  Port=2
  wires:
  Gain/1 -> gaze control/1
  gaze control/1 -> Product/2
  Product/1 -> gazeCmd/1
  Saturation/1 -> Product/1
  Trigger/1 -> Saturation/1
  RN vert/1 -> calcLoc vert x/y/5(beta)
  RN horiz/1 -> "calcLoc hor x/z "/5(beta)
  Mux/1 -> Add1/2
  "calcLoc hor x/z "/1(ndx) -> Add/1
  calcLoc vert x/y/2(ndy) -> gazelocation/2, Mux/2
  Add/1 -> Mux/1
  calcLoc vert x/y/1(ndx) -> Add/2
  "calcLoc hor x/z "/2(ndz) -> gazelocation/1, Mux/3
  Demux2/2 -> calcLoc vert x/y/4(y2)
  Demux1/2 -> calcLoc vert x/y/2(y1)
  Demux2/3 -> "calcLoc hor x/z "/4(z2)
  Demux2/1 -> calcLoc vert x/y/3(x2), "calcLoc hor x/z "/3(x2)
  Demux1/3 -> "calcLoc hor x/z "/2(z1)
  Demux1/1 -> calcLoc vert x/y/1(x1), "calcLoc hor x/z "/1(x1)
  "Speaker Position 3D "/1 -> Demux2/1
  Ego Position 3D/1 -> Demux1/1, Add1/1
  Demux/3 -> gaze control/3
  Demux/2 -> gaze control/2
  Demux/1 -> Gain/1
  extent/1 -> gaze control/4
  Add1/1 -> Demux/1, gazelocation1/1, Display/1

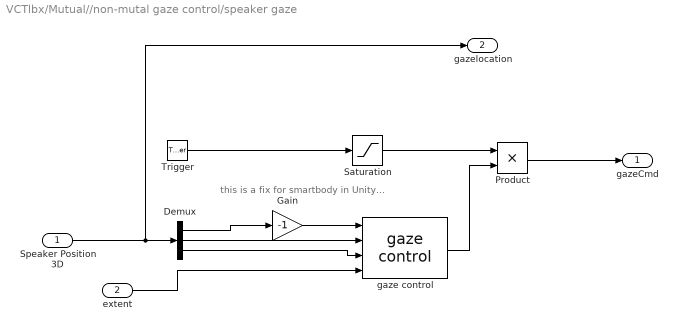
== system VCTlbx/Mutual//non-mutal gaze control/speaker gaze ==
  note: this is a fix for smartbody in Unity...
  "Speaker Position 3D " : Inport
  extent : Inport  Port=2
  Trigger : TriggerPort  TriggerType=either  VariantControl=Variant  ShowOutputPort=on
  Demux : Demux  Outputs=3
  Gain : Gain  Gain=-1
  Product : Product
  Saturation : Saturate  UpperLimit=1  LowerLimit=0
  gaze control : $bdroot/gaze control  SFunctionModules=''
  gazeCmd : Outport
  gazelocation : Outport  Port=2
  wires:
  Gain/1 -> gaze control/1
  gaze control/1 -> Product/2
  Product/1 -> gazeCmd/1
  Saturation/1 -> Product/1
  Trigger/1 -> Saturation/1
  "Speaker Position 3D "/1 -> Demux/1, gazelocation/1
  Demux/3 -> gaze control/3
  Demux/2 -> gaze control/2
  Demux/1 -> Gain/1
  extent/1 -> gaze control/4

== system VCTlbx/Poisson pulse/triggered Poisson ==
  Trigger : TriggerPort  VariantControl=Variant  PortDimensions=1
  Poisson numbers : commrandsrc3/Poisson Integer Generator  PoissonParameter=PoissonParameter  SeedSource=Auto  Seed=0  SampleTime=-1  SamplesPerFrame=1  OutputDataType=double  SimulateUsing=Interpreted execution
      settings: SourceProductName=Communications System Toolbox  SourceProductBaseCode=CM
  Scope : Scope  Commented=on
  delay : Outport
  wires:
  Poisson numbers/1 -> delay/1, Scope/1

== system VCTlbx/Mutual//non-mutal gaze control/Poisson social Gaze/p mutual ==
  Trigger : TriggerPort  TriggerType=either  VariantControl=Variant  ShowOutputPort=on  PortDimensions=1
  Display : Display
  Poisson numbers mutual : commrandsrc3/Poisson Integer Generator  PoissonParameter=PoissonParameterMutual  SeedSource=Auto  Seed=0  SampleTime=-1  SamplesPerFrame=1  OutputDataType=double  SimulateUsing=Interpreted execution
      settings: SourceProductName=Communications System Toolbox  SourceProductBaseCode=CM
  Product : Product
  Saturation : Saturate  UpperLimit=inf  LowerLimit=0
  lower: 0.5 : Saturate  UpperLimit=inf  LowerLimit=0.5
  delay : Outport
  wires:
  lower: 0.5/1 -> Product/2, Display/1
  Product/1 -> delay/1
  Saturation/1 -> Product/1
  Trigger/1 -> Saturation/1
  Poisson numbers mutual/1 -> lower: 0.5/1

== system VCTlbx/Mutual//non-mutal gaze control/Poisson social Gaze/p nonmutual ==
  Trigger : TriggerPort  TriggerType=either  VariantControl=Variant  ShowOutputPort=on  PortDimensions=1
  Poisson numbers nonmutual : commrandsrc3/Poisson Integer Generator  PoissonParameter=PoissonParameterNonMutual  SeedSource=Auto  Seed=0  SampleTime=-1  SamplesPerFrame=1  OutputDataType=double  SimulateUsing=Interpreted execution
      settings: SourceProductName=Communications System Toolbox  SourceProductBaseCode=CM
  Product : Product
  Saturation : Saturate  UpperLimit=inf  LowerLimit=0
  lower: 0.5 : Saturate  UpperLimit=inf  LowerLimit=0.5
  delay : Outport
  wires:
  lower: 0.5/1 -> Product/2
  Product/1 -> delay/1
  Saturation/1 -> Product/1
  Trigger/1 -> Saturation/1
  Poisson numbers nonmutual/1 -> lower: 0.5/1

== matlab function VCTlbx/3D coordinate transform/Y/MATLAB Function ==
  data: zeroA input; zeroB input; minmaxA input; minmaxB input; valA input; valB output
function valB = coordTrans(zeroA, zeroB, minmaxA, minmaxB, valA)
%#codegen
%coordinate transformation
% input:
% - min, max, zero 
% - min', max', zero' 
% zeroA = 0;
minA = minmaxA(1); %-1
maxA = minmaxA(2); %1;
%valA = -.5;
% zeroB = 0;
minB = minmaxB(1); %-10;
maxB = minmaxB(2); %10;

min_ratio = abs(zeroB-minB)/abs(zeroA-minA);
max_ratio = abs(zeroB-maxB)/abs(zeroA-maxA);
zero_shift=zeroB-zeroA;
if valA < zeroA
    valB = valA*min_ratio + zero_shift;
else
    valB = valA*max_ratio + zero_shift;
end

== matlab function VCTlbx/3D coordinate transform/X/MATLAB Function ==
  data: zeroA input; zeroB input; minmaxA input; minmaxB input; valA input; valB output
function valB = coordTrans(zeroA, zeroB, minmaxA, minmaxB, valA)
%#codegen
%coordinate transformation
% input:
% - min, max, zero 
% - min', max', zero' 
% zeroA = 0;
minA = minmaxA(1); %-1
maxA = minmaxA(2); %1;
%valA = -.5;
% zeroB = 0;
minB = minmaxB(1); %-10;
maxB = minmaxB(2); %10;

min_ratio = abs(zeroB-minB)/abs(zeroA-minA);
max_ratio = abs(zeroB-maxB)/abs(zeroA-maxA);
zero_shift=zeroB-zeroA;
if valA < zeroA
    valB = valA*min_ratio + zero_shift;
else
    valB = valA*max_ratio + zero_shift;
end

== matlab function VCTlbx/3D coordinate transform/Z/MATLAB Function ==
  data: zeroA input; zeroB input; minmaxA input; minmaxB input; valA input; valB output
function valB = coordTrans(zeroA, zeroB, minmaxA, minmaxB, valA)
%#codegen
%coordinate transformation
% input:
% - min, max, zero 
% - min', max', zero' 
% zeroA = 0;
minA = minmaxA(1); %-1
maxA = minmaxA(2); %1;
%valA = -.5;
% zeroB = 0;
minB = minmaxB(1); %-10;
maxB = minmaxB(2); %10;

min_ratio = abs(zeroB-minB)/abs(zeroA-minA);
max_ratio = abs(zeroB-maxB)/abs(zeroA-maxA);
zero_shift=zeroB-zeroA;
if valA < zeroA
    valB = valA*min_ratio + zero_shift;
else
    valB = valA*max_ratio + zero_shift;
end

== matlab function VCTlbx/conc msg ==
  data: y output; u1 input; u2 input
function y = fcn(u1, u2)
arr1 = double(deblank(char(u1')));
arr2 = double(deblank(char(u2')));
y = encStr2Arr(horzcat(arr1, arr2));

== matlab function VCTlbx/conc msg vector ==
  data: y output; u input
function y = fcn(u)
%coder.varsize('y', [2048, 1], [0 0])
%muxing create a concatenated vector....
u2 = reshape(u,2048,[]);
s = size(u2,2);

%size(u)
st = 1;
arr = zeros(1,2048);
for i=1:s
    slice=deblank(char(u2(:,i)'));
    cs=size(slice,2);
    t = double(slice);
    if(st+cs-1<=2048)
        arr(1, st:st+cs-1) = t; % coder does not like a=horzcat(a,t)....
    end
    st = st+cs;
end
y = encStr2Arr(arr);

== matlab function VCTlbx/createMessage ==
  data: y output; msg parameter
function y = fcn(msg)
y = msg;

== matlab function VCTlbx/facial Expressions/FEAnger ==
  data: ampl input; AU4 output; AU5 output; AU7 output; AU23 output
function[AU4, AU5, AU7, AU23] = fcn(ampl)
%AU1=ampl*-.8;
%AU2=ampl*1;
AU4=ampl*1;
AU5=ampl*1;
AU7=ampl*0.9;
AU23=ampl*1;
end

== matlab function VCTlbx/facial Expressions/FEDisgust ==
  data: ampl input; AU9 output; AU15 output; AU16 output
function[AU9, AU15, AU16] = fcn(ampl)
%AU9=ampl*0.9;
%AU10=ampl*0.1;
%AU17=ampl*0.7;
%wikipedia says: 9+15+16
AU9=ampl*1;
AU15=ampl*1;
AU16=ampl*1;

end

== matlab function VCTlbx/facial Expressions/FEFear ==
  data: ampl input; AU1 output; AU2 output; AU4 output; AU5 output; AU7 output; AU20 output; AU26 output
function[AU1, AU2, AU4, AU5, AU7, AU20, AU26] = fcn(ampl)
%function[AU1, AU2, AU4, AU5, AU20] = fcn(ampl)
%AU1=ampl*0.5;
%AU2=ampl*1;
%AU4=ampl*0.5;
%AU5=ampl*0.8;
%AU20=ampl*0.5;
 
%wikipedia says: 1+2+4+5+7+20+26
AU1=ampl*1;
AU2=ampl*1;
AU4=ampl*1;
AU5=ampl*1;
AU7=ampl*1;
AU20=ampl*1;
AU26=ampl*1;
end

== matlab function VCTlbx/facial Expressions/FEJoy ==
  data: ampl input; AU6 output; AU12 output
function [AU6, AU12] = fcn(ampl)
AU6=ampl*0.7;
AU12=ampl*0.8;
end

== matlab function VCTlbx/facial Expressions/FESadness ==
  data: ampl input; AU1 output; AU4 output; AU15 output
function[AU1, AU4, AU15] = fcn(ampl)
AU1=ampl*.8;
AU2=ampl*-.8;
AU7=ampl*0.7;
AU11=ampl*1;

%wikipedia says: 1+4+15
AU1=ampl*1;
AU4=ampl*1;
AU15=ampl*1;
end

== matlab function VCTlbx/facial Expressions/FESurprise ==
  data: ampl input; AU1 output; AU2 output; AU5 output; AU26 output
function[AU1, AU2, AU5, AU26] = fcn(ampl)
AU1=ampl*0.5;
AU2=ampl*1;
AU5=ampl*1;
AU26=ampl*0.5;
end

== matlab function VCTlbx/Add prefix//suffix ==
  data: y output; u input; prefix parameter; suffix parameter
function y = fcn(u, prefix, suffix)
%coder.varsize('y', [2048, 1], [0 0])
%muxing create a concatenated vector....
arr1 = double(deblank(char(prefix')));
arr2 = double(deblank(char(u')));
arr3 = double(deblank(char(suffix')));
y = encStr2Arr(horzcat(arr1, arr2, arr3));

== matlab function VCTlbx/Mutual//non-mutal gaze control/randomGaze/calcLoc hor x//z  ==
  data: ndx output; x1 input; ndz output; z1 input; x2 input; z2 input; beta input
function [ndx, ndz] = fcn(x1, z1, x2, z2, beta)
%#codegen
%beta=-pi/2;
dx = x2-x1;
dz = z2-z1;
h = sqrt(dz^2 + dx^2);
gamma = asin(dx/h) - pi/2 + beta;
alpha=(gamma*360)/(2*pi);
ndz = sin(gamma) * h;
ndx = cos(gamma) * h;

== matlab function VCTlbx/Mutual//non-mutal gaze control/randomGaze/calcLoc vert x//y ==
  data: x1 input; ndx output; y1 input; x2 input; y2 input; ndy output; beta input
function [ndx, ndy] = fcn(x1, y1, x2, y2, beta)
%#codegen
%beta=0;
dx = x2-x1;
dy = y2-y1;
h = sqrt(dx^2 + dy^2);
gamma = asin(dy/h) + beta;
ndx = cos(gamma) * h;
ndy = sin(gamma) * h;

== matlab function VCTlbx/Mutual//non-mutal gaze control/conc msg ==
  data: y output; u1 input; u2 input
function y = fcn(u1, u2)
arr1 = double(deblank(char(u1')));
arr2 = double(deblank(char(u2')));
y = encStr2Arr(horzcat(arr1, arr2));

== matlab function VCTlbx/facial Expressions CHL/FEAnger ==
  data: ampl input; AU4 output; AU5 output; AU7 output; AU23 output
function[AU4, AU5, AU7, AU23] = fcn(ampl)
%AU1=ampl*-.8;
%AU2=ampl*1;
AU4=ampl*1;
AU5=ampl*1;
AU7=ampl*0.9;
AU23=ampl*1;
end

== matlab function VCTlbx/facial Expressions CHL/FEDisgust ==
  data: ampl input; AU9 output; AU15 output; AU16 output
function[AU9, AU15, AU16] = fcn(ampl)
%AU9=ampl*0.9;
%AU10=ampl*0.1;
%AU17=ampl*0.7;
%wikipedia says: 9+15+16
AU9=ampl*1;
AU15=ampl*1;
AU16=ampl*1;

end

== matlab function VCTlbx/facial Expressions CHL/FEFear ==
  data: ampl input; AU1 output; AU2 output; AU4 output; AU5 output; AU7 output; AU20 output; AU26 output
function[AU1, AU2, AU4, AU5, AU7, AU20, AU26] = fcn(ampl)
%function[AU1, AU2, AU4, AU5, AU20] = fcn(ampl)
%AU1=ampl*0.5;
%AU2=ampl*1;
%AU4=ampl*0.5;
%AU5=ampl*0.8;
%AU20=ampl*0.5;
 
%wikipedia says: 1+2+4+5+7+20+26
AU1=ampl*1;
AU2=ampl*1;
AU4=ampl*1;
AU5=ampl*1;
AU7=ampl*1;
AU20=ampl*1;
AU26=ampl*1;
end

== matlab function VCTlbx/facial Expressions CHL/FEJoy ==
  data: ampl input; AU6 output; AU12 output
function [AU6, AU12] = fcn(ampl)
AU6=ampl*0.7;
AU12=ampl*0.8;
end

== matlab function VCTlbx/facial Expressions CHL/FESadness ==
  data: ampl input; AU1 output; AU4 output; AU15 output
function[AU1, AU4, AU15] = fcn(ampl)
AU1=ampl*.8;
AU2=ampl*-.8;
AU7=ampl*0.7;
AU11=ampl*1;

%wikipedia says: 1+4+15
AU1=ampl*1;
AU4=ampl*1;
AU15=ampl*1;
end

== matlab function VCTlbx/facial Expressions CHL/FESurprise ==
  data: ampl input; AU1 output; AU2 output; AU5 output; AU26 output
function[AU1, AU2, AU5, AU26] = fcn(ampl)
AU1=ampl*0.5;
AU2=ampl*1;
AU5=ampl*1;
AU26=ampl*0.5;
end
